simulink model "quadratic2006simulation"  (R2022b)
settings: Solver=VariableStepAuto  StartTime=0.0  StopTime=10.0  RelTol=1e-3
StartFcn:
  | run('quadratic2006parameters.m');
settings Model: Creator=kaganakar  LastModifiedBy=kaganakar

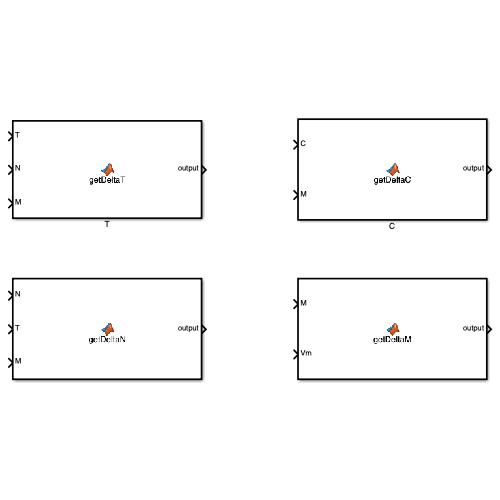
[thumbnail: Simulink's stored preview of the top-level diagram]
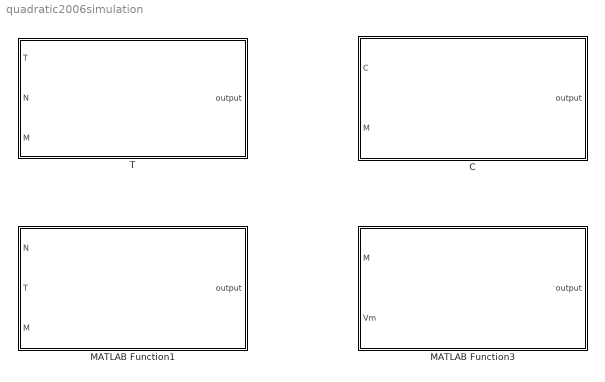
== system quadratic2006simulation ==
  C : MATLAB Function  TreatAsAtomicUnit=on
  MATLAB Function1 : MATLAB Function  TreatAsAtomicUnit=on
  MATLAB Function3 : MATLAB Function  TreatAsAtomicUnit=on
  T : MATLAB Function  TreatAsAtomicUnit=on

== matlab function quadratic2006simulation/MATLAB Function1 ==
  data: N input; T input; output output; M input
function output = getDeltaN(N,T,M)
    output = alpha1-f*N+g*(T)/(h+T)*N - p*N*T - kn*M*N;
end

== matlab function quadratic2006simulation/T ==
  data: T input; output output; N input; M input
function output = getDeltaT(T,N, M)
    output = a*T*(1-b*T)-c*N*T - kt*M*T;
end

== matlab function quadratic2006simulation/C ==
  data: C input; output output; M input
function output = getDeltaC(C,M)
    output = alpha2 - beta*C - kc*M*C;
end

== matlab function quadratic2006simulation/MATLAB Function3 ==
  data: M input; Vm input; output output
function output = getDeltaM(M, Vm)
    output = -gamma*M + Vm;
end
